simulink model "simulation"  (R2016a)
settings: Solver=ode14x  SolverMode=SingleTasking  StartTime=0.0  StopTime=sim_time_sec  FixedStep=h  RelTol=1e-3
undefined symbols (not defined in the file): cm_to_rad, Gamma, h, initial_state, K, K_c, K_m, Phi, sim_time_sec, step_size_cm
libraries: simulink x1
settings Model: Creator=robin  LastModifiedBy=robin
settings DataIOCC: ReturnWorkspaceOutputs=on
settings DebuggingCC: UnconnectedInputMsg=none  UnconnectedOutputMsg=none  UnconnectedLineMsg=none  SFUnexpectedBacktrackingDiag=error  SFNoUnconditionalDefaultTransitionDiag=error
settings ModelReferenceCC: EnableRefExpFcnMdlSchedulingChecks=off
settings SFSimCC: SimUseLocalCustomCode=on
settings RTWCC: Description=Generic Real-Time Target  RTWUseLocalCustomCode=on
settings GRTTargetCC: TargetLangStandard=C99 (ISO)
settings ConfigComp: CovMetricSettings=dwe  CovSaveCumulativeToWorkspaceVar=off  CovSaveSingleToWorkspaceVar=off  CovExternalEMLEnable=on

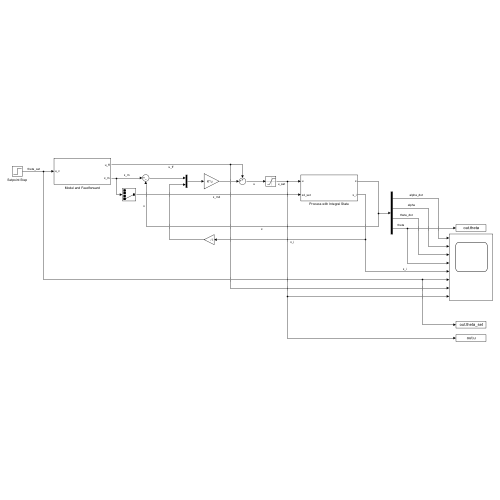
[thumbnail: Simulink's stored preview of the top-level diagram]
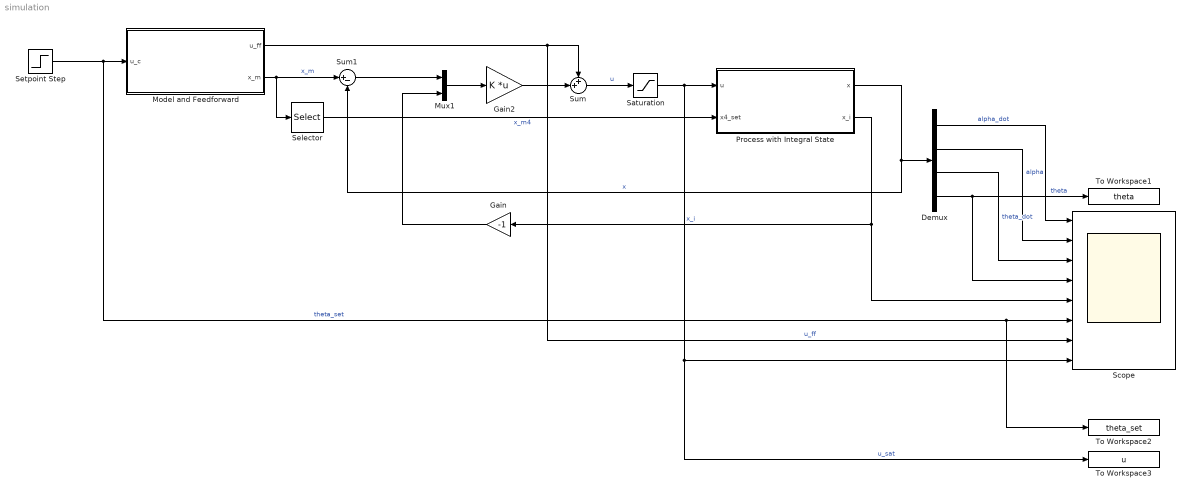
== system simulation ==
  Demux : Demux
  Gain : Gain  Gain=-1
  Gain2 : Gain  Gain=K  Multiplication=Matrix(K*u)
  Model and Feedforward : Subsystem
  Mux1 : Mux  Inputs=2
  Process with Integral State : Subsystem
  Saturation : Saturate  UpperLimit=9  LowerLimit=-9
  Scope : Scope  NumInputPorts=8
  Selector : Selector  InputPortWidth=4  IndexOptions=Index vector (dialog)  Indices=4  OutputSizes=1
  Setpoint Step : Step  Time=sim_time_sec / 4  After=step_size_cm * cm_to_rad  SampleTime=h
  Sum : Sum  Inputs=++|
  Sum1 : Sum  Inputs=|+-
  To Workspace1 : ToWorkspace  VariableName=theta  SaveFormat=Timeseries  SampleTime=-1
  To Workspace2 : ToWorkspace  VariableName=theta_set  SaveFormat=Timeseries  SampleTime=-1
  To Workspace3 : ToWorkspace  VariableName=u  SaveFormat=Timeseries  SampleTime=-1
  wires:
  Setpoint Step/1 -> Scope/6, To Workspace2/1, Model and Feedforward/1(u_c)  "theta_set"
  Gain2/1 -> Sum/2
  Demux/1 -> Scope/1  "alpha_dot"
  Demux/2 -> Scope/2  "alpha"
  Demux/3 -> Scope/3  "theta_dot"
  Demux/4 -> Scope/4, To Workspace1/1  "theta"
  Process with Integral State/1(x) -> Sum1/2, Demux/1  "x"
  Sum1/1 -> Mux1/1
  Model and Feedforward/2(x_m) -> Selector/1, Sum1/1  "x_m"
  Model and Feedforward/1(u_ff) -> Scope/7, Sum/1  "u_ff"
  Saturation/1 -> Process with Integral State/1(u), Scope/8, To Workspace3/1  "u_sat"
  Sum/1 -> Saturation/1  "u"
  Process with Integral State/2(x_i) -> Scope/5, Gain/1  "x_i"
  Mux1/1 -> Gain2/1
  Gain/1 -> Mux1/2
  Selector/1 -> Process with Integral State/2(x4_set)  "x_m4"

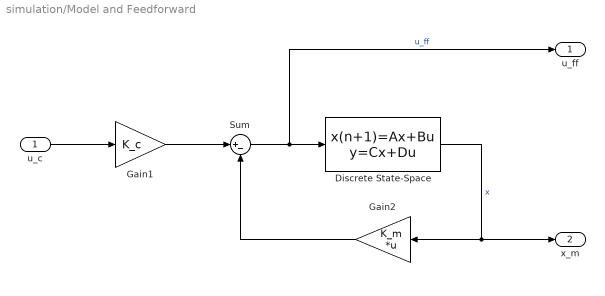
== system simulation/Model and Feedforward ==
  u_c : Inport
  Discrete State-Space : DiscreteStateSpace  A=Phi  B=Gamma  C=eye(size(Phi))  D=zeros(size(Phi, 1), 1)  SampleTime=-1  StateIdentifier={'alpha_dot', 'alpha', 'theta_dot', 'theta', 'x_i'}
  Gain1 : Gain  Gain=K_c
  Gain2 : Gain  Gain=K_m  Multiplication=Matrix(K*u)
  Sum : Sum  Inputs=|+-
  u_ff : Outport
  x_m : Outport  Port=2
  wires:
  Discrete State-Space/1 -> x_m/1, Gain2/1  "x"
  u_c/1 -> Gain1/1
  Gain1/1 -> Sum/1
  Sum/1 -> u_ff/1, Discrete State-Space/1  "u_ff"
  Gain2/1 -> Sum/2

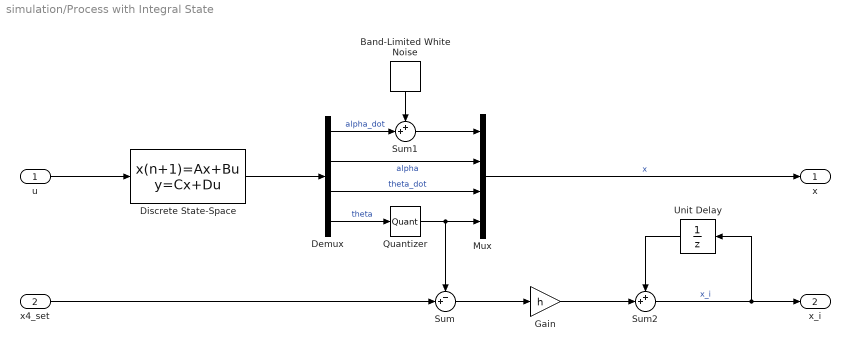
== system simulation/Process with Integral State ==
  u : Inport
  x4_set : Inport  Port=2
  Band-Limited White Noise : simulink/Sources/Band-Limited White Noise  Cov=[0.002]  Ts=0.2  seed=[23341]
  Demux : Demux
  Discrete State-Space : DiscreteStateSpace  A=Phi  B=Gamma  C=eye(size(Phi))  D=zeros(size(Phi, 1), 1)  X0=initial_state(1:end-1)  SampleTime=-1  StateIdentifier={'alpha_dot', 'alpha', 'theta_dot', 'theta', 'x_i'}
  Gain : Gain  Gain=h
  Mux : Mux
  Quantizer : Quantizer  QuantizationInterval=deg2rad(0.5)
  Sum : Sum  Inputs=-+|
  Sum1 : Sum  Inputs=++|
  Sum2 : Sum  Inputs=++|
  Unit Delay : UnitDelay  InitialCondition=initial_state(5)  SampleTime=-1  HasFrameUpgradeWarning=on
  x : Outport
  x_i : Outport  Port=2
  wires:
  Discrete State-Space/1 -> Demux/1
  u/1 -> Discrete State-Space/1
  Demux/1 -> Sum1/2  "alpha_dot"
  Demux/2 -> Mux/2  "alpha"
  Demux/3 -> Mux/3  "theta_dot"
  Demux/4 -> Quantizer/1  "theta"
  Quantizer/1 -> Sum/1, Mux/4
  Band-Limited White Noise/1 -> Sum1/1
  Sum1/1 -> Mux/1
  Mux/1 -> x/1  "x"
  x4_set/1 -> Sum/2
  Unit Delay/1 -> Sum2/1
  Sum/1 -> Gain/1
  Sum2/1 -> Unit Delay/1, x_i/1  "x_i"
  Gain/1 -> Sum2/2
